simulink model "SimulacionControl2017a"  (R2017a)
settings: Solver=VariableStepAuto  StartTime=0.0  StopTime=fin  FixedStep=0.001  RelTol=1e-3
values from neighbouring files (symbols this model uses):
  Ts_control = 0.001    [A_SimulacionAnalisis.m]
undefined symbols (not defined in the file or in its folder): mcd
undefined symbols (not defined in the file): mci
libraries: dspsrcs4 x3
settings Model: Creator=Richa  LastModifiedBy=richard

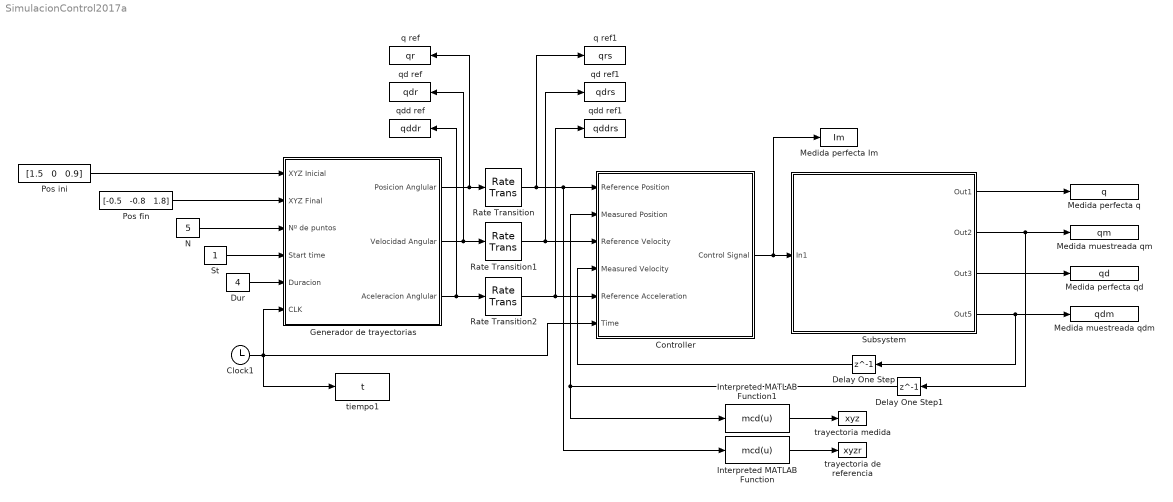
== system SimulacionControl2017a ==
  Clock1 : Clock
  Controller : Subsystem  TreatAsAtomicUnit=on  SystemSampleTime=Ts_control
      mask DialogControl Control2 Prompt: Controller
  Delay One Step : Delay  DelayLength=1
  Delay One Step1 : Delay  DelayLength=1
  Dur : Constant  Value=4
  Generador de trayectorias : Subsystem
      mask Display: image('screenshot.png');
  Interpreted MATLAB Function : MATLABFcn  MATLABFcn=mcd(u)
  Interpreted MATLAB Function1 : MATLABFcn  MATLABFcn=mcd(u)
  Medida muestreada qdm : ToWorkspace  VariableName=qdm  SampleTime=Ts_control
  Medida muestreada qm : ToWorkspace  VariableName=qm  SampleTime=Ts_control
  Medida perfecta Im : ToWorkspace  VariableName=Im
  Medida perfecta q : ToWorkspace  VariableName=q  SampleTime=-1
  Medida perfecta qd : ToWorkspace  VariableName=qd  SampleTime=-1
  N : Constant  Value=5
  Pos fin : Constant  Value="[-0.5   -0.8   1.8]"
  Pos ini : Constant  Value="[1.5   0   0.9]"
  Rate Transition : RateTransition  OutPortSampleTimeMultiple=ZOH  OutPortSampleTime=Ts_reference
  Rate Transition1 : RateTransition  OutPortSampleTime=Ts_reference
  Rate Transition2 : RateTransition  OutPortSampleTime=Ts_reference
  St : Constant
  Subsystem : Subsystem
  q ref : ToWorkspace  VariableName=qr  SampleTime=-1
  q ref1 : ToWorkspace  VariableName=qrs
  qd ref : ToWorkspace  VariableName=qdr  SampleTime=-1
  qd ref1 : ToWorkspace  VariableName=qdrs
  qdd ref : ToWorkspace  VariableName=qddr  SampleTime=-1
  qdd ref1 : ToWorkspace  VariableName=qddrs
  tiempo1 : ToWorkspace  VariableName=t
  trayectoria de referencia : ToWorkspace  VariableName=xyzr
  trayectoria medida : ToWorkspace  VariableName=xyz
  wires:
  Pos fin/1 -> Generador de trayectorias/2(XYZ Final)
  Pos ini/1 -> Generador de trayectorias/1(XYZ Inicial)
  St/1 -> Generador de trayectorias/4(Start time)
  N/1 -> Generador de trayectorias/3(Nº de puntos)
  Dur/1 -> Generador de trayectorias/5(Duracion)
  Clock1/1 -> tiempo1/1, Controller/6(Time), Generador de trayectorias/6(CLK)
  Controller/1(Control Signal) -> Medida perfecta Im/1, Subsystem/1(In1)
  Generador de trayectorias/1(" Posicion Anglular") -> Rate Transition/1, q ref/1
  Generador de trayectorias/2(Velocidad Angular) -> Rate Transition1/1, qd ref/1
  Generador de trayectorias/3(Aceleracion Anglular) -> Rate Transition2/1, qdd ref/1
  Rate Transition1/1 -> Controller/3(Reference Velocity), qd ref1/1
  Rate Transition2/1 -> Controller/5(Reference Acceleration), qdd ref1/1
  Interpreted MATLAB Function/1 -> trayectoria de referencia/1
  Rate Transition/1 -> Interpreted MATLAB Function/1, Controller/1(Reference Position), q ref1/1
  Interpreted MATLAB Function1/1 -> trayectoria medida/1
  Subsystem/3(Out3) -> Medida perfecta qd/1
  Subsystem/1(Out1) -> Medida perfecta q/1
  Subsystem/4(Out5) -> Delay One Step/1, Medida muestreada qdm/1
  Subsystem/2(Out2) -> Delay One Step1/1, Medida muestreada qm/1
  Delay One Step1/1 -> Controller/2(Measured Position), Interpreted MATLAB Function1/1
  Delay One Step/1 -> Controller/4(Measured Velocity)

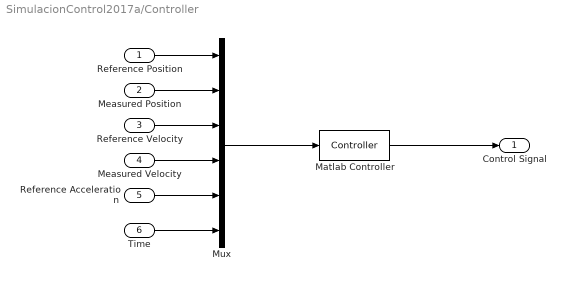
== system SimulacionControl2017a/Controller ==
  Reference Position : Inport
  Measured Position : Inport  Port=2
  Reference Velocity : Inport  Port=3
  Measured Velocity : Inport  Port=4
  Reference Acceleration : Inport  Port=5
  Time : Inport  Port=6
  "Matlab Controller " : MATLABFcn  MATLABFcn=Controller  OutputDimensions=3
  Mux : Mux  Inputs=6
  Control Signal : Outport
  wires:
  Reference Velocity/1 -> Mux/3
  Reference Acceleration/1 -> Mux/5
  Reference Position/1 -> Mux/1
  Measured Position/1 -> Mux/2
  Measured Velocity/1 -> Mux/4
  Mux/1 -> "Matlab Controller "/1
  Time/1 -> Mux/6
  "Matlab Controller "/1 -> Control Signal/1

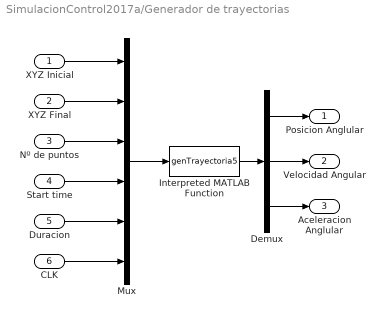
== system SimulacionControl2017a/Generador de trayectorias ==
  XYZ Inicial : Inport
  XYZ Final : Inport  Port=2
  Nº de puntos : Inport  Port=3
  Start time : Inport  Port=4
  Duracion : Inport  Port=5
  CLK : Inport  Port=6
  Demux : Demux  Outputs=3
  Interpreted MATLAB Function : MATLABFcn  MATLABFcn=genTrayectoria5  OutputDimensions=9
  Mux : Mux  Inputs=6
  " Posicion Anglular" : Outport  PortDimensions=3
  Velocidad Angular : Outport  Port=2  PortDimensions=3
  Aceleracion Anglular : Outport  Port=3  PortDimensions=3
  wires:
  Demux/3 -> Aceleracion Anglular/1
  Mux/1 -> Interpreted MATLAB Function/1
  Nº de puntos/1 -> Mux/3
  CLK/1 -> Mux/6
  Start time/1 -> Mux/4
  Interpreted MATLAB Function/1 -> Demux/1
  Duracion/1 -> Mux/5
  XYZ Final/1 -> Mux/2
  XYZ Inicial/1 -> Mux/1
  Demux/1 -> " Posicion Anglular"/1
  Demux/2 -> Velocidad Angular/1

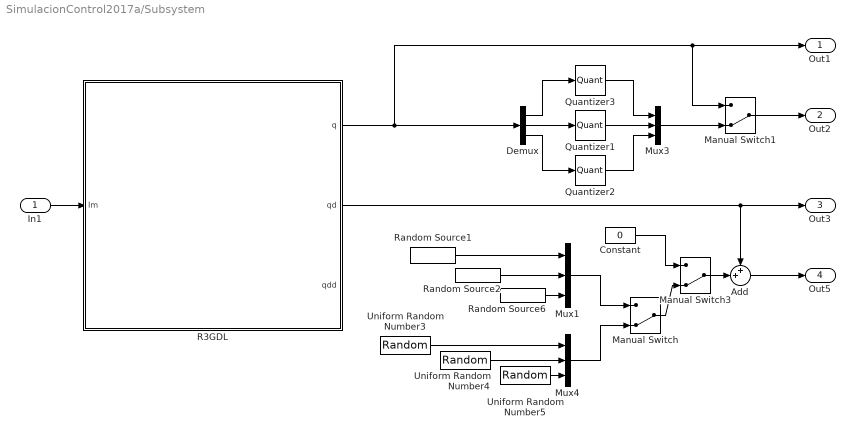
== system SimulacionControl2017a/Subsystem ==
  In1 : Inport
  Add : Sum  Inputs=++|
  Constant : Constant  Value=0
  Demux : Demux  Outputs=3
  Manual Switch : ManualSwitch  CurrentSetting=0
  Manual Switch1 : ManualSwitch  CurrentSetting=0
  Manual Switch3 : ManualSwitch  CurrentSetting=0
  Mux1 : Mux  Inputs=3
  Mux3 : Mux  Inputs=3
  Mux4 : Mux  Inputs=3
  Quantizer1 : Quantizer  QuantizationInterval=2*pi/1024/30
  Quantizer2 : Quantizer  QuantizationInterval=2*pi/1024/15
  Quantizer3 : Quantizer  QuantizationInterval=2*pi/1024/50
  R3GDL : Subsystem  mask(Control y Programación de Robots (4 GIERM)){NGrupo=15, q1_ini=[1 0 0]*mci([1.5   0   0.9],1), q2_ini=[0 1 0]*mci([1.5   0   0.9],1), q3_ini=[0 0 1]*mci([1.5   0   0.9],1), Bl_q1=off, Bl_q2=off, Bl_q3=off, AccionamientoDirecto=on}
      mask prompts: NGrupo "Nº de GRUPO"; q1_ini "q1 inicial  (rad)"; q2_ini "q2 inicial (rad)"; q3_ini "q3_inicial (rad)"; Bl_q1 "Bloqueo q1"; Bl_q2 "Bloqueo q2"; Bl_q3 "Bloqueo q3"; AccionamientoDirecto "Accionamiento directo"
      mask help: Robot de 3 grados de libertad RRR
      mask Display:
      | image(imread('R3GDL_RRR.JPG'));
      | port_label('output', 1, 'q');
      | port_label('output', 2, 'qd');
      | port_label('output', 3, 'qdd');
      | port_label('input', 1, 'Im')
  Random Source1 : dspsrcs4/Random Source  SrcType=Uniform  NormMethod=Ziggurat  CltLength=12  MinVal=-(1500*2*pi/60)*(0.01/50)  MaxVal=(1500*2*pi/60)*(0.01/50)  MeanVal=0  VarVal=1  RepMode=Not repeatable  rawSeed=1  IsInherit=off  SampMode=Continuous  SampTime=1  SampFrame=1  DataType=Double  OutComplex=Real  OutputFrames=off
  Random Source2 : dspsrcs4/Random Source  SrcType=Uniform  NormMethod=Ziggurat  CltLength=12  MinVal=-(1500*2*pi/60)*(0.01/30)  MaxVal=(1500*2*pi/60)*(0.01/30)  MeanVal=0  VarVal=1  RepMode=Not repeatable  rawSeed=1  IsInherit=off  SampMode=Continuous  SampTime=1  SampFrame=1  DataType=Double  OutComplex=Real  OutputFrames=off
  Random Source6 : dspsrcs4/Random Source  SrcType=Uniform  NormMethod=Ziggurat  CltLength=12  MinVal=-(1500*2*pi/60)*(0.01/15)  MaxVal=(1500*2*pi/60)*(0.01/15)  MeanVal=0  VarVal=1  RepMode=Not repeatable  rawSeed=1  IsInherit=off  SampMode=Continuous  SampTime=1  SampFrame=1  DataType=Double  OutComplex=Real  OutputFrames=off
  Uniform Random Number3 : UniformRandomNumber  Minimum=-(1500*2*pi/60)*(0.01/50)  Maximum=(1500*2*pi/60)*(0.01/50)  SampleTime=0.001
  Uniform Random Number4 : UniformRandomNumber  Minimum=-(1500*2*pi/60)*(0.01/30)  Maximum=(1500*2*pi/60)*(0.01/30)  SampleTime=0.001
  Uniform Random Number5 : UniformRandomNumber  Minimum=-(1500*2*pi/60)*(0.01/15)  Maximum=(1500*2*pi/60)*(0.01/15)  SampleTime=0.001
  Out1 : Outport
  Out2 : Outport  Port=2
  Out3 : Outport  Port=3
  Out5 : Outport  Port=4
  wires:
  In1/1 -> R3GDL/1(Im)
  R3GDL/2(qd) -> Add/1, Out3/1
  Add/1 -> Out5/1
  Quantizer2/1 -> Mux3/3
  Demux/1 -> Quantizer3/1
  Quantizer1/1 -> Mux3/2
  Demux/3 -> Quantizer2/1
  Quantizer3/1 -> Mux3/1
  Demux/2 -> Quantizer1/1
  Random Source6/1 -> Mux1/3
  Random Source2/1 -> Mux1/2
  Random Source1/1 -> Mux1/1
  R3GDL/1(q) -> Demux/1, Manual Switch1/1, Out1/1
  Mux1/1 -> Manual Switch/1
  Mux4/1 -> Manual Switch/2
  Manual Switch1/1 -> Out2/1
  Mux3/1 -> Manual Switch1/2
  Uniform Random Number3/1 -> Mux4/1
  Uniform Random Number4/1 -> Mux4/2
  Uniform Random Number5/1 -> Mux4/3
  Manual Switch/1 -> Manual Switch3/2
  Manual Switch3/1 -> Add/2
  Constant/1 -> Manual Switch3/1

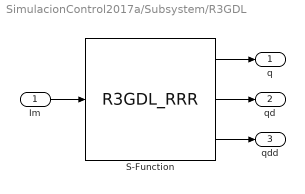
== system SimulacionControl2017a/Subsystem/R3GDL ==
  Im : Inport
  S-Function : S-Function  FunctionName=R3GDL_RRR  Parameters=[q1_ini; q2_ini; q3_ini]; [Bl_q1; Bl_q2; Bl_q3]; AccionamientoDirecto; NGrupo  SFunctionDeploymentMode=off  EnableBusSupport=off
  q : Outport
  qd : Outport  Port=2
  qdd : Outport  Port=3
  wires:
  Im/1 -> S-Function/1
  S-Function/1 -> q/1
  S-Function/2 -> qd/1
  S-Function/3 -> qdd/1
